simulink model "Heli_OpenLoop"  (Simulink 6.3)
settings: Solver=ode1  SolverMode=SingleTasking  StartTime=0.0  StopTime=inf  FixedStep=0.001  RelTol=1e-3
values from neighbouring files (symbols this model uses):
  JOYSTICK_X_DZ = 0.25    [setup_heli_LQR_instructor.m]    (also in setup_heli_LQR_parameters.m)
  JOYSTICK_Y_DZ = 0.25    [setup_heli_LQR_instructor.m]    (also in setup_heli_LQR_parameters.m)
  K_CABLE_P = 5    [setup_heli_LQR_instructor.m]    (also in setup_heli_LQR_parameters.m)
  K_CABLE_Y = 3    [setup_heli_LQR_instructor.m]    (also in setup_heli_LQR_parameters.m)
  K_EC_P = - 2 * pi / ( 4 * 1024 )    (= -0.00153398078789)    [setup_heli_LQR_instructor.m]    (also in setup_heli_LQR_parameters.m)
  K_EC_Y = 2 * pi / ( 8 * 1024 )    (= 0.000766990393943)    [setup_heli_LQR_instructor.m]    (also in setup_heli_LQR_parameters.m)
  theta_0 = -30*pi/180    (= -0.523598775598)    [setup_heli_LQR_instructor.m]    (also in setup_heli_LQR_parameters.m)
  VMAX_DAC = 10    [setup_heli_LQR_instructor.m]    (also in setup_heli_LQR_parameters.m)
  VMAX_UPM_P = 24    [setup_heli_LQR_instructor.m]    (also in setup_heli_LQR_parameters.m)
  VMAX_UPM_Y = 15    [setup_heli_LQR_instructor.m]    (also in setup_heli_LQR_parameters.m)
  Vpe = 9    [setup_heli_LQR_instructor.m]    (also in setup_heli_LQR_parameters.m)
  Vye = -9    [setup_heli_LQR_instructor.m]    (also in setup_heli_LQR_parameters.m)
  wcf = 2 * pi * 20    (= 125.663706144)    [setup_heli_LQR_instructor.m]    (also in setup_heli_LQR_parameters.m)
  zetaf = 0.85    [setup_heli_LQR_instructor.m]    (also in setup_heli_LQR_parameters.m)
undefined symbols (not defined in the file or in its folder): Joystick, q_modules3
libraries: qctools x3
settings Model: LastModifiedBy=localadmin  ExtModeArmWhenConnect=off  BufferReuse=off  StrictBusMsg=None
settings ConfigSet: SimulationMode=external
settings OptimizationCC: BooleanDataType=off  InlineInvariantSignals=on  OptimizeBlockIOStorage=off  BufferReuse=off  ExpressionFolding=off  LocalBlockOutputs=off
settings RTWCC: SystemTargetFile=wincon.tlc  MakeCommand=make_wc  TemplateMakefile=wc_default_tmf  Description=WinCon Target  ProcessScript=wincon_make_rtw_hook
settings STFCustomTargetCC: TargetFcnLib=ansi_tfl_tmw.mat  GenFloatMathFcnCalls=ANSI_C  ModelReferenceCompliant=off  SystemTargetFile=wincon.tlc
settings GRTTargetCC: ModelReferenceCompliant=off  MatFileLogging=off  ExtMode=on  ExtModeTransport=2  ExtModeMexFile=wc_comm
settings CustomProperty: Value=on

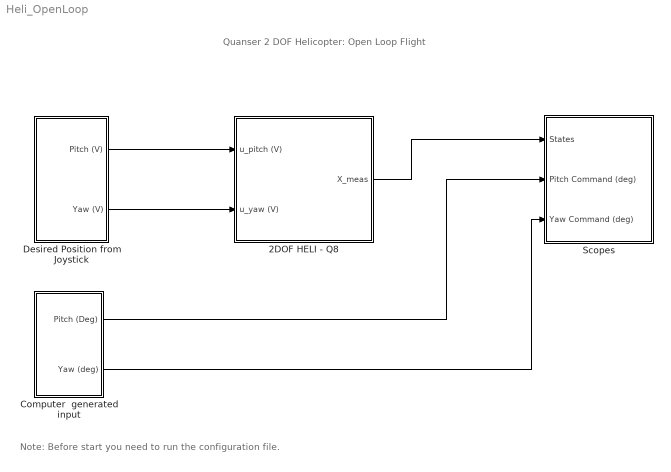
== system Heli_OpenLoop ==
  note: Quanser 2 DOF Helicopter:
      | Open Loop Flight
  note: Note: Before start you need to run the configuration file.
  2DOF HELI - Q8 : Subsystem  AncestorBlock=heli_2d_lib/2DOF HELI - Q8
  Computer  generated input : Subsystem
  Desired Position from Joystick : Subsystem  AncestorBlock=q_modules3/Joystick
  Scopes : Subsystem
  wires:
  2DOF HELI - Q8/1(X_meas) -> Scopes/1(States)
  Desired Position from Joystick/1(Pitch (V)) -> 2DOF HELI - Q8/1(u_pitch (V))
  Desired Position from Joystick/2(Yaw (V)) -> 2DOF HELI - Q8/2(u_yaw (V))
  Computer  generated input/1(Pitch (Deg)) -> Scopes/2(Pitch Command (deg))
  Computer  generated input/2(Yaw (deg)) -> Scopes/3(Yaw Command (deg))

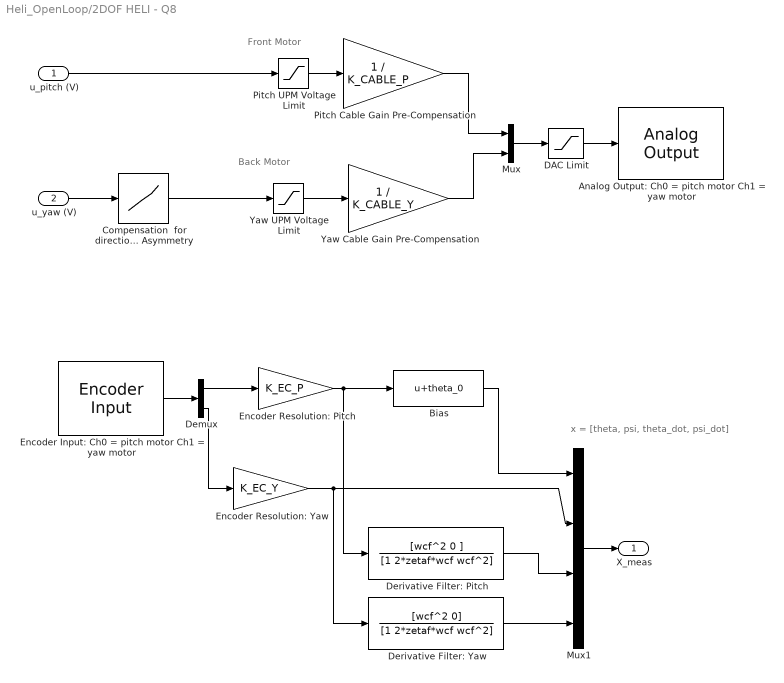
== system Heli_OpenLoop/2DOF HELI - Q8 ==
  note: Back Motor
  note: Front Motor
  note: x = [theta, psi, theta_dot, psi_dot]
  u_pitch (V) : Inport
  u_yaw (V) : Inport  Port=2
  Analog Output: Ch0 = pitch motor Ch1 = yaw motor : qctools/Quanser Consulting Q8 Series/Analog Output  boardNumber=0  channels=[0,1]  modesVect=0  rangesVect=10  initialVect=0  finalVect=0  sampleTime=-1  inputVolts=on  simulationOutput=off
  Bias : Bias  Bias=theta_0
  "Compensation  for direction Asymmetry " : Lookup  InputValues="[-[12.5  10 7.5]  0  [7.5 10  12.5 15] ]"  OutputValues="[-[12.5  10 7.5] *.4 0  [7.5 10  12.5 15] ]"
  DAC Limit : Saturate  UpperLimit=VMAX_DAC  LowerLimit=- VMAX_DAC
  Demux : Demux  Outputs=2
  Derivative Filter: Pitch : TransferFcn  Numerator=[wcf^2 0 ]  Denominator=[1 2*zetaf*wcf wcf^2]
  Derivative Filter: Yaw : TransferFcn  Numerator=[wcf^2 0]  Denominator=[1 2*zetaf*wcf wcf^2]
  Encoder Input: Ch0 = pitch motor Ch1 = yaw motor : qctools/Quanser Consulting Q8 Series/Encoder Input  boardNumber=0  channels=[0,1]  initial=0  preserveCounts=off  sampleTime=default_sample_time  quadratureStr=4X  modeStr=Normal  flagString=FLG1 is IDX and FLG2 is E  prescale=1  frequency=16666666.6667  bcd=off  enableIndex=on  synchronousIndex=on  indexPolarity=on  reloadOnIndex=off  simulationInput=off
  "Encoder Resolution: Pitch " : Gain  Gain=K_EC_P
  Encoder Resolution: Yaw : Gain  Gain=K_EC_Y
  Mux : Mux  Inputs=2
  Mux1 : Mux
  Pitch Cable Gain Pre-Compensation : Gain  Gain=1 / K_CABLE_P  SaturateOnIntegerOverflow=on
  Pitch UPM Voltage Limit : Saturate  UpperLimit=VMAX_UPM_P  LowerLimit=- VMAX_UPM_P
  Yaw Cable Gain Pre-Compensation : Gain  Gain=1 / K_CABLE_Y  SaturateOnIntegerOverflow=on
  Yaw UPM Voltage Limit : Saturate  UpperLimit=VMAX_UPM_Y  LowerLimit=- VMAX_UPM_Y
  X_meas : Outport
  wires:
  Encoder Resolution: Yaw/1 -> Mux1/2, Derivative Filter: Yaw/1
  Yaw Cable Gain Pre-Compensation/1 -> Mux/2
  Pitch Cable Gain Pre-Compensation/1 -> Mux/1
  Mux1/1 -> X_meas/1
  u_pitch (V)/1 -> Pitch UPM Voltage Limit/1
  Yaw UPM Voltage Limit/1 -> Yaw Cable Gain Pre-Compensation/1
  Pitch UPM Voltage Limit/1 -> Pitch Cable Gain Pre-Compensation/1
  DAC Limit/1 -> Analog Output: Ch0 = pitch motor Ch1 = yaw motor/1
  Mux/1 -> DAC Limit/1
  Demux/1 -> "Encoder Resolution: Pitch "/1
  "Encoder Resolution: Pitch "/1 -> Bias/1, Derivative Filter: Pitch/1
  Encoder Input: Ch0 = pitch motor Ch1 = yaw motor/1 -> Demux/1
  Demux/2 -> Encoder Resolution: Yaw/1
  Bias/1 -> Mux1/1
  Derivative Filter: Pitch/1 -> Mux1/3
  Derivative Filter: Yaw/1 -> Mux1/4
  "Compensation  for direction Asymmetry "/1 -> Yaw UPM Voltage Limit/1
  u_yaw (V)/1 -> "Compensation  for direction Asymmetry "/1

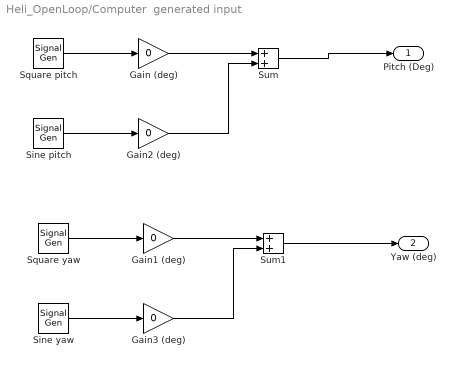
== system Heli_OpenLoop/Computer  generated input ==
  Gain (deg) : Gain  Gain=0
  Gain1 (deg) : Gain  Gain=0
  Gain2 (deg) : Gain  Gain=0
  Gain3 (deg) : Gain  Gain=0
  Sine pitch : SignalGenerator  Frequency=1/30
  Sine yaw : SignalGenerator  Frequency=.02
  Square pitch : SignalGenerator  WaveForm=square  Frequency=1/30
  Square yaw : SignalGenerator  WaveForm=square  Frequency=1/60*2
  Sum : Sum
  Sum1 : Sum
  Pitch (Deg) : Outport
  Yaw (deg) : Outport  Port=2
  wires:
  Gain3 (deg)/1 -> Sum1/2
  Sine yaw/1 -> Gain3 (deg)/1
  Sum1/1 -> Yaw (deg)/1
  Gain1 (deg)/1 -> Sum1/1
  Square yaw/1 -> Gain1 (deg)/1
  Gain2 (deg)/1 -> Sum/2
  Sine pitch/1 -> Gain2 (deg)/1
  Sum/1 -> Pitch (Deg)/1
  Gain (deg)/1 -> Sum/1
  Square pitch/1 -> Gain (deg)/1

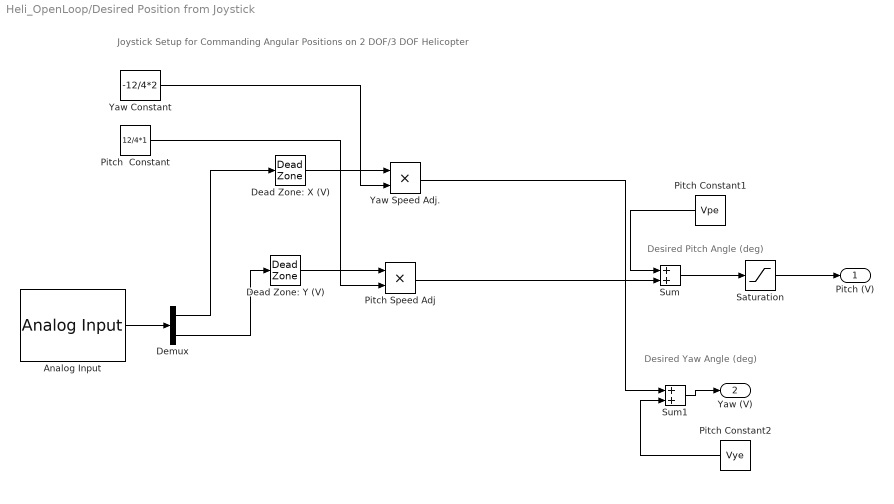
== system Heli_OpenLoop/Desired Position from Joystick ==
  note: Joystick Setup for Commanding Angular Positions on 2 DOF/3 DOF Helicopter
  note: Desired Yaw Angle (deg)
  note: Desired Pitch Angle (deg)
  Analog Input : qctools/Quanser Consulting Q8 Series/Analog Input  boardNumber=0  channels=[2 3]  sampleTime=default_sample_time  useBusy=on  simultaneous=on  outputVolts=on  simulationInput=off
  Dead Zone: X (V) : DeadZone  LowerValue=-JOYSTICK_X_DZ  UpperValue=JOYSTICK_X_DZ  SaturateOnIntegerOverflow=on
  Dead Zone: Y (V) : DeadZone  LowerValue=-JOYSTICK_Y_DZ  UpperValue=JOYSTICK_Y_DZ  SaturateOnIntegerOverflow=on
  Demux : Demux  Outputs=2
  Pitch  Constant : Constant  Value=12/4*1
  Pitch Constant1 : Constant  Orientation=left  Value=Vpe
  Pitch Constant2 : Constant  Orientation=left  Value=Vye
  Pitch Speed Adj : Product  RndMeth=Zero
  Saturation : Saturate  UpperLimit=11  LowerLimit=2
  Sum : Sum
  Sum1 : Sum
  Yaw Constant : Constant  Value=-12/4*2
  Yaw Speed Adj. : Product  RndMeth=Zero
  Pitch (V) : Outport
  Yaw (V) : Outport  Port=2
  wires:
  Pitch  Constant/1 -> Pitch Speed Adj/2
  Demux/2 -> Dead Zone: Y (V)/1
  Demux/1 -> Dead Zone: X (V)/1
  Yaw Constant/1 -> Yaw Speed Adj./2
  Analog Input/1 -> Demux/1
  Pitch Speed Adj/1 -> Sum/2
  Yaw Speed Adj./1 -> Sum1/1
  Dead Zone: Y (V)/1 -> Pitch Speed Adj/1
  Dead Zone: X (V)/1 -> Yaw Speed Adj./1
  Sum/1 -> Saturation/1
  Pitch Constant1/1 -> Sum/1
  Pitch Constant2/1 -> Sum1/2
  Sum1/1 -> Yaw (V)/1
  Saturation/1 -> Pitch (V)/1

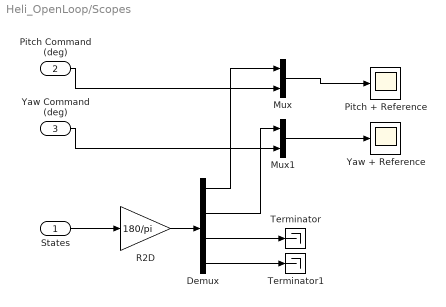
== system Heli_OpenLoop/Scopes ==
  States : Inport
  Pitch Command (deg) : Inport  Port=2
  Yaw Command (deg) : Inport  Port=3
  Demux : Demux
  Mux : Mux  Inputs=2
  Mux1 : Mux  Inputs=2
  Pitch + Reference : Scope
      settings: SaveName=ScopeData6
  R2D : Gain  Gain=180/pi
  Terminator : Terminator
  Terminator1 : Terminator
  Yaw + Reference : Scope
      settings: SaveName=ScopeData7
  wires:
  States/1 -> R2D/1
  R2D/1 -> Demux/1
  Mux/1 -> Pitch + Reference/1
  Mux1/1 -> Yaw + Reference/1
  Demux/3 -> Terminator/1
  Demux/4 -> Terminator1/1
  Demux/1 -> Mux/1
  Pitch Command (deg)/1 -> Mux/2
  Yaw Command (deg)/1 -> Mux1/2
  Demux/2 -> Mux1/1
